simulink model "test02_Select_From_Array"  (Simulink 7.4)
settings: Solver=ode3  StartTime=0.0  StopTime=10.0  FixedStep=0.0000000000001  RelTol=1e-3
libraries: NAV420Lib x1
settings Model: Creator=djulzz  LastModifiedBy=djulzz

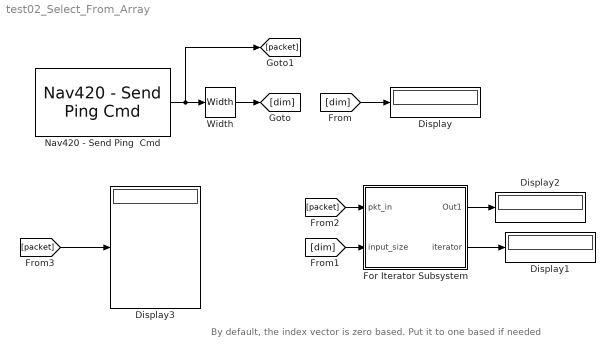
== system test02_Select_From_Array ==
  note: By default, the index vector is zero based. Put it to one based if needed
  Display{,1..3} (4 alike) : Display
      Display3 settings: Format=hex (Stored Integer)
  For Iterator Subsystem : Subsystem  TreatAsAtomicUnit=on
  Nav420 - Send Ping  Cmd : NAV420Lib/Nav420 - Send Ping  Cmd  SystemSampleTime=-1
  Width : Width
  wires:
  Nav420 - Send Ping  Cmd/1 -> Width/1, [packet]
  Width/1 -> [dim]
  [dim] -> Display/1
  [dim] -> For Iterator Subsystem/2(input_size)
  For Iterator Subsystem/2(iterator) -> Display1/1
  [packet] -> For Iterator Subsystem/1(pkt_in)
  For Iterator Subsystem/1(Out1) -> Display2/1
  [packet] -> Display3/1

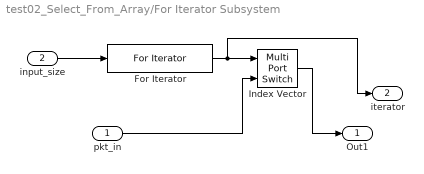
== system test02_Select_From_Array/For Iterator Subsystem ==
  pkt_in : Inport  OutDataType=fixdt(1, 16)  OutScaling=2^0
  input_size : Inport  Port=2  OutDataType=fixdt(1, 16)  OutScaling=2^0
  For Iterator : ForIterator  IterationSource=external
  Index Vector : MultiPortSwitch  Inputs=1  OutDataTypeMode=uint8  OutDataType=fixdt(1, 16)  OutScaling=2^0  OutDataTypeStr=uint8
  Out1 : Outport  DataType=uint8  OutDataType=fixdt(1, 16)  OutScaling=2^0  OutDataTypeStr=uint8
  iterator : Outport  Port=2  OutDataType=fixdt(1, 16)  OutScaling=2^0
  wires:
  input_size/1 -> For Iterator/1
  For Iterator/1 -> Index Vector/1, iterator/1
  pkt_in/1 -> Index Vector/2
  Index Vector/1 -> Out1/1
